simulink model "EKF_pendulum_random_walk"  (R2019b)
settings: Solver=FixedStepAuto  StartTime=0.0  StopTime=100  FixedStep=sim_freq  RelTol=1e-3
values from neighbouring files (symbols this model uses):
  b = 0.1    [myStateTransitionFcn.m]    (also in pendulum_EKF.m = 0.5; random_walk_pendulum_EKF.m)
  g = 9.81    [myStateTransitionFcn.m]    (also in pendulum_EKF.m; random_walk_pendulum_EKF.m)
  I = 0.1    [myStateTransitionFcn.m]    (also in pendulum_EKF.m = 2; random_walk_pendulum_EKF.m)
  L = 0.5    [myStateTransitionFcn.m]    (also in pendulum_EKF.m = 1; random_walk_pendulum_EKF.m)
  m = 1    [myStateTransitionFcn.m]    (also in pendulum_EKF.m = 2; random_walk_pendulum_EKF.m)
  meas_theta_dot_var = 0.0001    [pendulum_EKF.m]    (also in random_walk_pendulum_EKF.m = 1e-06)
  meas_theta_var = 0.0001    [pendulum_EKF.m]    (also in random_walk_pendulum_EKF.m = 1e-06)
  Pk_init = zeros(2)    [pendulum_EKF.m]    (also in random_walk_pendulum_EKF.m = zeros(3))
  Qk = C22'*C12    [pendulum_EKF.m]    (also in random_walk_pendulum_EKF.m; symbolic_pendulum_ekf.m = eye(2)*[process_theta_variance;process_theta_dot_variance]*T; symbolic_pendulum_random_walk_ekf.m = eye(2)*[process_theta_variance;process_theta_dot_variance]*T)
  Rk = [meas_theta_var 0; 0 meas_theta_dot_var]    [pendulum_EKF.m]    (also in random_walk_pendulum_EKF.m = [meas_theta_var 0 ; 0 meas_theta_dot_var])
  Ts = 0.004    [pendulum_EKF.m]    (also in random_walk_pendulum_EKF.m; symbolic_pendulum_ekf.m; symbolic_pendulum_random_walk_ekf.m)
  X_hat_init = [0;0]    [pendulum_EKF.m]    (also in random_walk_pendulum_EKF.m = [0;0;0])
libraries: sharedTrackingLibrary x1
settings Model: Creator=henry  LastModifiedBy=henry

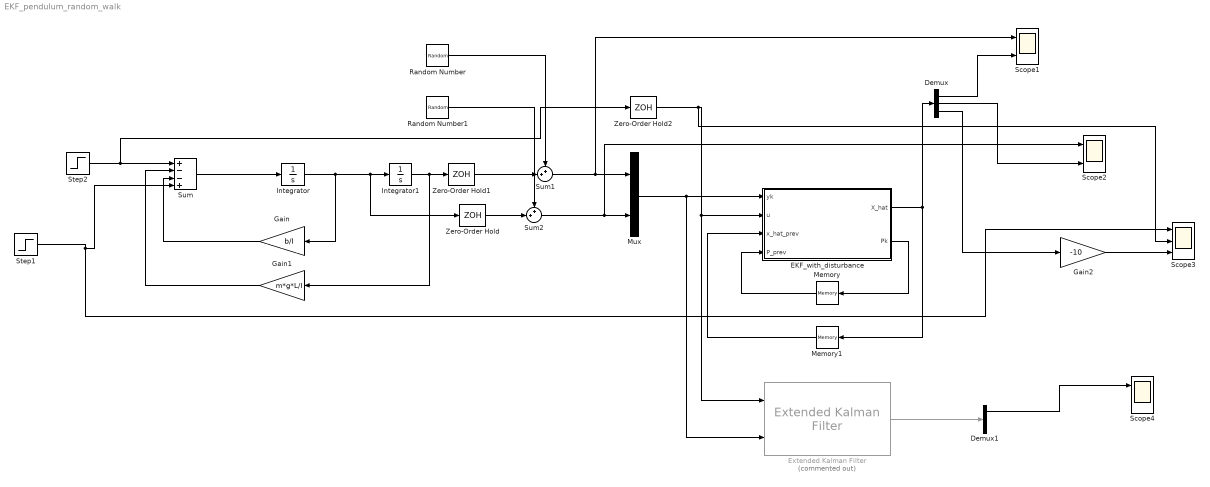
== system EKF_pendulum_random_walk ==
  Demux : Demux  Outputs=3
  Demux1 : Demux  Outputs=3
  EKF_with_disturbance : MATLAB Function  TreatAsAtomicUnit=on
  Extended Kalman Filter : sharedTrackingLibrary/Extended Kalman Filter  Commented=on  StateTransitionFcn=myStateTransitionFcn  HasStateTransitionJacobianFcn=off  HasAdditiveProcessNoise=Additive  ProcessNoise=Qk  HasTimeVaryingProcessNoise=off  HasStateTransitionFcnExtraArgument=1  InitialState=X_hat_init  InitialStateCovariance=Pk_init  MeasurementFcn1=myMeasurementFcn  HasMeasurementJacobianFcn1=off  HasMeasurementEnablePort1=off  HasAdditiveMeasurementNoise1=Additive  MeasurementNoise1=Rk  HasTimeVaryingMeasurementNoise1=off  HasMeasurementFcnExtraArgument1=0  MeasurementFcn2=myMeasurementFcn  HasMeasurementJacobianFcn2=off  HasMeasurementEnablePort2=off  HasAdditiveMeasurementNoise2=Additive  MeasurementNoise2=1  HasTimeVaryingMeasurementNoise2=off  HasMeasurementFcnExtraArgument2=0  MeasurementFcn3=myMeasurementFcn  HasMeasurementJacobianFcn3=off  HasMeasurementEnablePort3=off  HasAdditiveMeasurementNoise3=Additive  MeasurementNoise3=1  HasTimeVaryingMeasurementNoise3=off  HasMeasurementFcnExtraArgument3=0  MeasurementFcn4=myMeasurementFcn  HasMeasurementJacobianFcn4=off  HasMeasurementEnablePort4=off  HasAdditiveMeasurementNoise4=Additive  MeasurementNoise4=1  HasTimeVaryingMeasurementNoise4=off  HasMeasurementFcnExtraArgument4=0  MeasurementFcn5=myMeasurementFcn  HasMeasurementJacobianFcn5=off  HasMeasurementEnablePort5=off  HasAdditiveMeasurementNoise5=Additive  MeasurementNoise5=1  HasTimeVaryingMeasurementNoise5=off  HasMeasurementFcnExtraArgument5=0  EnableMultirate=off  StateTransitionFcnSampleTime=1  MeasurementFcn1SampleTime=1  MeasurementFcn2SampleTime=1  MeasurementFcn3SampleTime=1  MeasurementFcn4SampleTime=1  MeasurementFcn5SampleTime=1  UseCurrentEstimator=on  OutputStateCovariance=off  DataType=double  SampleTime=1  NumberOfMeasurements=1
      settings: SourceProductName=Automated Driving Toolbox  SourceProductBaseCode=DR
  Gain : Gain  Gain=b/I
  Gain1 : Gain  Gain=m*g*L/I
  Gain2 : Gain  Gain=-10
  Integrator : Integrator
  Integrator1 : Integrator
  Memory : Memory  InitialCondition=Pk_init
  Memory1 : Memory  InitialCondition=X_hat_init
  Mux : Mux  Inputs=2
  Random Number : RandomNumber  Variance=meas_theta_var  Seed=1  SampleTime=Ts
  Random Number1 : RandomNumber  Variance=meas_theta_dot_var  Seed=2  SampleTime=Ts
  Scope1 : Scope  NumInputPorts=2
  Scope2 : Scope  NumInputPorts=2
  Scope3 : Scope  NumInputPorts=3
  Scope4 : Scope  NumInputPorts=2
  Step1 : Step  Time=5  SampleTime=0
  Step2 : Step  Time=2  After=0  SampleTime=0
  Sum : Sum  Inputs=+--+
  Sum1 : Sum  Inputs=++|
  Sum2 : Sum  Inputs=++|
  Zero-Order Hold : ZeroOrderHold  SampleTime=Ts
  Zero-Order Hold1 : ZeroOrderHold  SampleTime=Ts
  Zero-Order Hold2 : ZeroOrderHold  SampleTime=Ts
  wires:
  Integrator/1 -> Gain/1, Zero-Order Hold/1, Integrator1/1
  Sum/1 -> Integrator/1
  Gain/1 -> Sum/3
  Gain1/1 -> Sum/2
  Random Number/1 -> Sum1/1
  Mux/1 -> Extended Kalman Filter/2, EKF_with_disturbance/1(yk)
  EKF_with_disturbance/2(Pk) -> Memory/1
  Memory/1 -> EKF_with_disturbance/4(P_prev)
  Memory1/1 -> EKF_with_disturbance/3(x_hat_prev)
  Integrator1/1 -> Gain1/1, Zero-Order Hold1/1
  Random Number1/1 -> Sum2/1
  Step2/1 -> Zero-Order Hold2/1, Sum/1
  Zero-Order Hold/1 -> Sum2/2
  Zero-Order Hold1/1 -> Sum1/2
  Sum2/1 -> Scope2/1, Mux/2
  EKF_with_disturbance/1(X_hat) -> Demux/1, Memory1/1
  Demux/2 -> Scope2/2
  Demux/1 -> Scope1/2
  Sum1/1 -> Scope1/1, Mux/1
  Step1/1 -> Scope3/1, Sum/4
  Gain2/1 -> Scope3/3
  Demux/3 -> Gain2/1
  Extended Kalman Filter/1 -> Demux1/1
  Demux1/1 -> Scope4/1
  Zero-Order Hold2/1 -> Extended Kalman Filter/1, EKF_with_disturbance/2(u), Scope3/2

== matlab function EKF_pendulum_random_walk/EKF_with_disturbance ==
  data: yk input size=[2 1]; u input; X_hat output size=[3 1]; x_hat_prev input size=[3 1]; P_prev input size=[3 3]; Pk output size=[3 3]; m parameter; g parameter; L parameter; I parameter; b parameter; Qk parameter size=[3 3]; Rk parameter size=[2 2]
function [X_hat,Pk]= fcn(yk,u,x_hat_prev,P_prev,m, g, L, I, b, Qk, Rk)


F1 = @(x,U) x(2);
F2 = @(x,U) U/I-(m*g*L/I)*sin( x(1) ) - x(2)*b/I - x(3)/I;
F3 = @(x,U) 0;
H1 = @(x) x(1);
H2 = @(x) x(2);


% Jacobian
Fk = @(x,U) [1, 1/250, 0;(-L*g*m)*cos( x(1) )/(250*I), 1 - b/(250*I), -1/(250*I); 0, 0, 1];



%% Control Update
Pk_ =  Fk(x_hat_prev,u) * P_prev * transpose( Fk(x_hat_prev,u) ) + Qk;
Xk_ = x_hat_prev + [ F1(x_hat_prev,u)*1/250; F2(x_hat_prev,u)*1/250; F3(x_hat_prev,u)*1/250]; 

Hk = [1 0 0; 0 1 0];

%% Measurement Update
Lk = Pk_*transpose(Hk)*inv(Hk*Pk_*transpose(Hk) + Rk);
Pk = (eye(3) - Lk*Hk)*Pk_;
X_hat = Xk_ + Lk*(yk - [ H1(Xk_);H2(Xk_)]);
